simulink model "ExtDem_SetPoint"  (R2016b)
settings: configuration reference "CodeGenConfigSet" (kept outside this file)
values from neighbouring files (symbols this model uses):
  EPM_N_ZERO = fi(0,EngSpeed_rpm)    [init_ExtDem_SetPoint.m]
  ExtDem_swtTrqSel_C = Calibration.Parameter    [init_ExtDem_SetPoint.m]
  ExtDem_tiTrqPT1_C = Calibration.Parameter    [init_ExtDem_SetPoint.m]
libraries: CXLib x2
settings Model: Creator=bianxuyin  LastModifiedBy=xuxingpei
settings ConfigSetRef: SourceLocation=Base Workspace

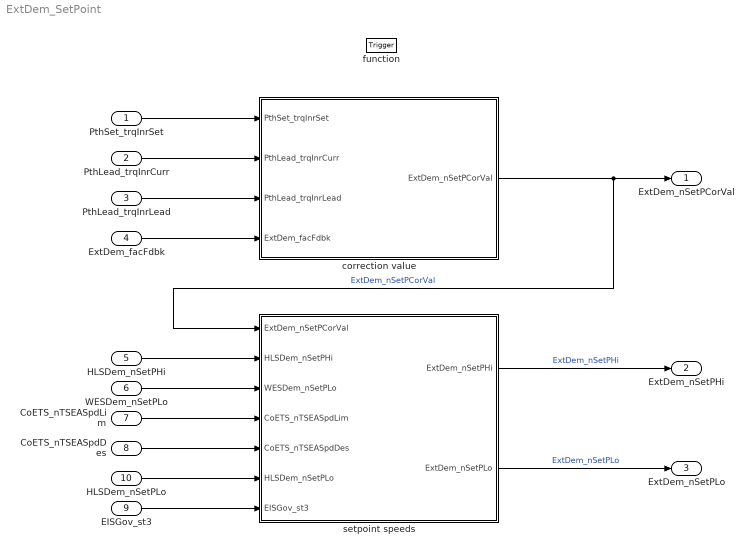
== system ExtDem_SetPoint ==
  PthSet_trqInrSet : Inport  Tag=Nm  Description=Inner torque set value after monitoring limitation  OutMin=-3000  OutMax=3276.7  OutDataTypeStr=Trq_Nm
  PthLead_trqInrCurr : Inport  Tag=Nm  Description=Actual percent engine torque  Port=2  OutMin=-3000  OutMax=3000  OutDataTypeStr=Trq_Nm
  PthLead_trqInrLead : Inport  Tag=Nm  Description=Inner torque lead value  Port=3  OutMin=-3000  OutMax=3000  OutDataTypeStr=Trq_Nm
  ExtDem_facFdbk : Inport  Tag=rpm/Nm  Description=External intervention feedback factor  Port=4  OutMin=-20  OutMax=20  OutDataTypeStr=FdbkNm2rpm_rpm_Nm
  HLSDem_nSetPHi : Inport  Tag=rpm  Description=Maximum engine speed of HLSDem  Port=5  OutMin=0  OutMax=6000  OutDataTypeStr=EngSpeed_rpm
  WESDem_nSetPLo : Inport  Tag=rpm  Description=Lower setpoint speed interval of WESDem  Port=6  OutMin=0  OutMax=6000  OutDataTypeStr=EngSpeed_rpm
  CoETS_nTSEASpdLim : Inport  Tag=rpm  Description=|  Port=7  OutMin=0  OutMax=6000  OutDataTypeStr=EngSpeed_rpm
      | The engine speed limitation requested from TSC1
      | CAN messages. This engine speed limit is given to
      | the speed governor
  CoETS_nTSEASpdDes : Inport  Tag=rpm  Description=The desired/control engine speed requested from TSC1 CAN messages. This desired/control engine speed is given to the speed governor.  Port=8  OutMin=0  OutMax=6000  OutDataTypeStr=EngSpeed_rpm
  EISGov_st3 : Inport  Description=Status information of WESDem client  Port=9  OutMin=0  OutMax=2147483648  OutDataTypeStr=State_uint32
  HLSDem_nSetPLo : Inport  Tag=rpm  Description=Minimum engine speed of HLSDem  Port=10  OutMin=0  OutMax=6000  OutDataTypeStr=EngSpeed_rpm
  function : TriggerPort  TriggerType=function-call  VariantControl=Variant
  " correction value" : Subsystem
  setpoint speeds : Subsystem
  ExtDem_nSetPCorVal : Outport  Tag=rpm  Description=Setpoint for correction factor calculation  OutMin=0  OutMax=6000  OutDataTypeStr=EngSpeed_rpm
  ExtDem_nSetPHi : Outport  Tag=rpm  Description=Higher limit of external demand set point speed  Port=2  OutMin=0  OutMax=6000  OutDataTypeStr=EngSpeed_rpm
  ExtDem_nSetPLo : Outport  Tag=rpm  Description=Lower limit of external demand set point speed  Port=3  OutMin=0  OutMax=6000  OutDataTypeStr=EngSpeed_rpm
  wires:
  " correction value"/1(ExtDem_nSetPCorVal) -> setpoint speeds/1(ExtDem_nSetPCorVal), ExtDem_nSetPCorVal/1  "ExtDem_nSetPCorVal"
  PthSet_trqInrSet/1 -> " correction value"/1(PthSet_trqInrSet)
  PthLead_trqInrCurr/1 -> " correction value"/2(PthLead_trqInrCurr)
  PthLead_trqInrLead/1 -> " correction value"/3(PthLead_trqInrLead)
  ExtDem_facFdbk/1 -> " correction value"/4(ExtDem_facFdbk)
  setpoint speeds/1(ExtDem_nSetPHi) -> ExtDem_nSetPHi/1  "ExtDem_nSetPHi"
  setpoint speeds/2(ExtDem_nSetPLo) -> ExtDem_nSetPLo/1  "ExtDem_nSetPLo"
  WESDem_nSetPLo/1 -> setpoint speeds/3(WESDem_nSetPLo)
  CoETS_nTSEASpdLim/1 -> setpoint speeds/4(CoETS_nTSEASpdLim)
  HLSDem_nSetPHi/1 -> setpoint speeds/2(HLSDem_nSetPHi)
  EISGov_st3/1 -> setpoint speeds/7(EISGov_st3)
  CoETS_nTSEASpdDes/1 -> setpoint speeds/5(CoETS_nTSEASpdDes)
  HLSDem_nSetPLo/1 -> setpoint speeds/6(HLSDem_nSetPLo)

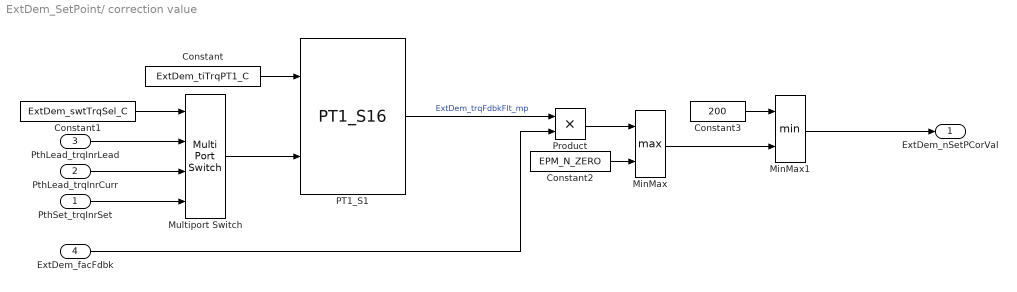
== system ExtDem_SetPoint/ correction value ==
  PthSet_trqInrSet : Inport  Tag=Nm  Description=Inner torque set value after monitoring limitation  OutMin=-3000  OutMax=3276.7  OutDataTypeStr=Trq_Nm
  PthLead_trqInrCurr : Inport  Tag=Nm  Description=Actual percent engine torque  Port=2  OutMin=-3000  OutMax=3000  OutDataTypeStr=Trq_Nm
  PthLead_trqInrLead : Inport  Tag=Nm  Description=Inner torque lead value  Port=3  OutMin=-3000  OutMax=3000  OutDataTypeStr=Trq_Nm
  ExtDem_facFdbk : Inport  Description=External intervention feedback factor  Port=4  OutMin=-20  OutMax=20  OutDataTypeStr=FdbkNm2rpm_rpm_Nm
  Constant : Constant  Value=ExtDem_tiTrqPT1_C
  Constant1 : Constant  Value=ExtDem_swtTrqSel_C
  Constant2 : Constant  Value=EPM_N_ZERO
  Constant3 : Constant  Value=200  OutDataTypeStr=Inherit: Inherit via back propagation
  MinMax : MinMax  Function=max  Inputs=2  InputSameDT=on
  MinMax1 : MinMax  Inputs=2  OutMin=0  OutMax=200  OutDataTypeStr=Inherit: Inherit via back propagation  InputSameDT=on
  Multiport Switch : MultiPortSwitch  DataPortOrder=Specify indices  DataPortIndices={2,1,0}  SaturateOnIntegerOverflow=on  InputSameDT=on
  PT1_S1 : CXLib/PT1_S16
  Product : Product  OutDataTypeStr=Inherit: Inherit via back propagation
  ExtDem_nSetPCorVal : Outport  Tag=rpm  Description=Setpoint for correction factor calculation  OutMin=0  OutMax=6000  OutDataTypeStr=EngSpeed_rpm
  wires:
  PT1_S1/1 -> Product/1  "ExtDem_trqFdbkFlt_mp"
  ExtDem_facFdbk/1 -> Product/2
  Constant/1 -> PT1_S1/1
  PthSet_trqInrSet/1 -> Multiport Switch/4
  PthLead_trqInrCurr/1 -> Multiport Switch/3
  PthLead_trqInrLead/1 -> Multiport Switch/2
  Constant1/1 -> Multiport Switch/1
  Multiport Switch/1 -> PT1_S1/2
  Product/1 -> MinMax/1
  Constant2/1 -> MinMax/2
  MinMax/1 -> MinMax1/2
  MinMax1/1 -> ExtDem_nSetPCorVal/1
  Constant3/1 -> MinMax1/1

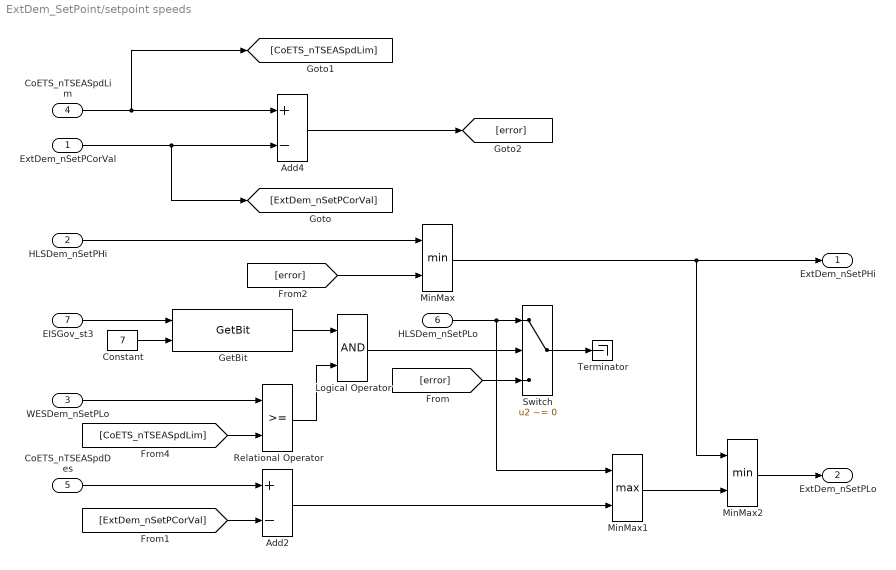
== system ExtDem_SetPoint/setpoint speeds ==
  ExtDem_nSetPCorVal : Inport  Tag=rpm  Description=Minimum engine speed of HLSDem  OutMin=0  OutMax=6000  OutDataTypeStr=EngSpeed_rpm
  HLSDem_nSetPHi : Inport  Tag=rpm  Description=Minimum engine speed of HLSDem  Port=2  OutMin=0  OutMax=6000  OutDataTypeStr=EngSpeed_rpm
  WESDem_nSetPLo : Inport  Tag=rpm  Description=Lower setpoint speed interval of WESDem  Port=3  OutMin=0  OutMax=6000  OutDataTypeStr=EngSpeed_rpm
  CoETS_nTSEASpdLim : Inport  Tag=rpm  Description=The engine speed limitation requested from TSC1 CAN messages. This engine speed limit is given to the speed governor.  Port=4  OutMin=-16384  OutMax=16383.5  OutDataTypeStr=EngSpeed_rpm
  CoETS_nTSEASpdDes : Inport  Tag=rpm  Description=The desired/control engine speed requested from TSC1 CAN messages. This desired/control engine speed is given to the speed governor.  Port=5  OutMin=0  OutMax=6000  OutDataTypeStr=EngSpeed_rpm
  HLSDem_nSetPLo : Inport  Tag=rpm  Description=Minimum engine speed of HLSDem  Port=6  OutMin=0  OutMax=6000  OutDataTypeStr=EngSpeed_rpm
  EISGov_st3 : Inport  Description=Status information of WESDem client  Port=7  OutMin=0  OutMax=2147483648  OutDataTypeStr=State_uint32
  Add2 : Sum  Inputs=+-  InputSameDT=on
  Add4 : Sum  Inputs=+-  SaturateOnIntegerOverflow=on  InputSameDT=on
  Constant : Constant  Value=7  OutDataTypeStr=Inherit: Inherit via back propagation
  GetBit : CXLib/GetBit  dataTypeString=uint32  dataLength=0
      settings: AttributesFormatString=Get bit from %<dataTypeString>
  Logical Operator : Logic  AllPortsSameDT=off  OutDataTypeStr=boolean
  MinMax : MinMax  Inputs=2  InputSameDT=on
  MinMax1 : MinMax  Function=max  Inputs=2  InputSameDT=on
  MinMax2 : MinMax  Inputs=2  InputSameDT=on
  Relational Operator : RelationalOperator  OutDataTypeStr=boolean  RndMeth=Simplest
  Switch : Switch  Criteria=u2 ~= 0  InputSameDT=on
  Terminator : Terminator
  ExtDem_nSetPHi : Outport  Tag=rpm  Description=Higher limit of external demand set point speed  OutMin=0  OutMax=6000  OutDataTypeStr=EngSpeed_rpm
  ExtDem_nSetPLo : Outport  Tag=rpm  Description=Lower limit of external demand set point speed  Port=2  OutMin=0  OutMax=6000  OutDataTypeStr=EngSpeed_rpm
  wires:
  HLSDem_nSetPHi/1 -> MinMax/1
  EISGov_st3/1 -> GetBit/1
  Constant/1 -> GetBit/2
  CoETS_nTSEASpdDes/1 -> Add2/1
  GetBit/1 -> Logical Operator/1
  [ExtDem_nSetPCorVal] -> Add2/2
  WESDem_nSetPLo/1 -> Relational Operator/1
  [CoETS_nTSEASpdLim] -> Relational Operator/2
  Logical Operator/1 -> Switch/2
  HLSDem_nSetPLo/1 -> MinMax1/1, Switch/1
  Relational Operator/1 -> Logical Operator/2
  MinMax/1 -> MinMax2/1, ExtDem_nSetPHi/1
  MinMax1/1 -> MinMax2/2
  MinMax2/1 -> ExtDem_nSetPLo/1
  Add2/1 -> MinMax1/2
  ExtDem_nSetPCorVal/1 -> Add4/2, [ExtDem_nSetPCorVal]
  CoETS_nTSEASpdLim/1 -> Add4/1, [CoETS_nTSEASpdLim]
  Add4/1 -> [error]
  [error] -> MinMax/2
  [error] -> Switch/3
  Switch/1 -> Terminator/1
